simulink model "fullMF"  (R2023b)
settings: Solver=VariableStepAuto  StartTime=0.0  StopTime=3000/fs  RelTol=1e-3
values from neighbouring files (symbols this model uses):
  fs = 16e6    (= 16000000)    [FullMF_startup.m]    (also in MF_startup.m)
  template11 = part11-part21    [FullMF_startup.m]
  template12 = part12-part22    [FullMF_startup.m]
  template13 = part13-part23    [FullMF_startup.m]
  template14 = part14-part24    [FullMF_startup.m]
  template21 = part31+part41    [FullMF_startup.m]
  template22 = part32+part42    [FullMF_startup.m]
  template23 = part33+part43    [FullMF_startup.m]
  template24 = part34+part44    [FullMF_startup.m]
undefined symbols (not defined in the file or in its folder): exp_W1, exp_W2, exp_W3, exp_W4
libraries: hdlBasic x200, hdlDSPIP x20, hdlsllib x1, vmcUtilities x1
(part 2 of 2)

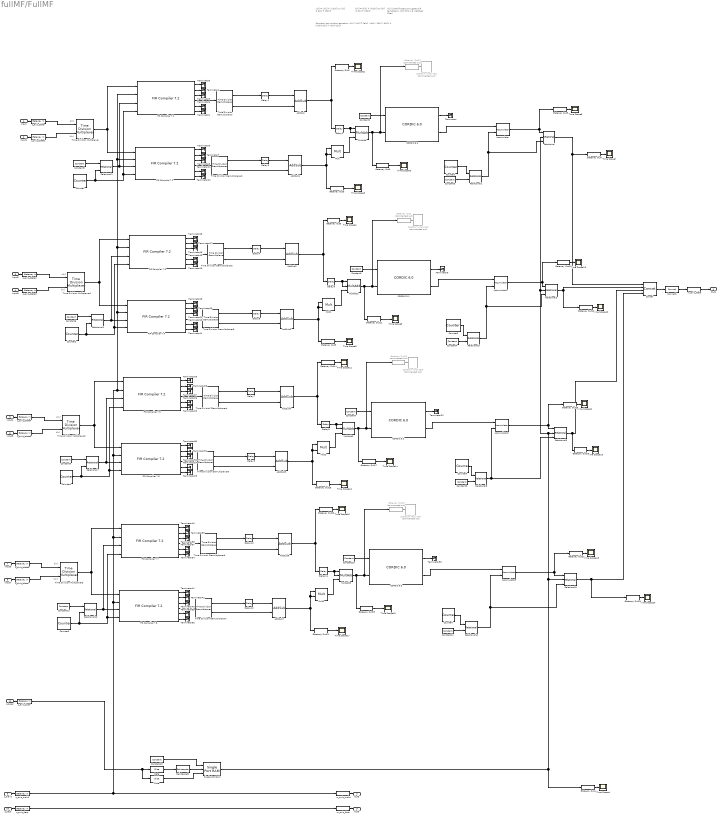
== system fullMF/FullMF ==
  note: a[n]
  note: b[n]
  note: x[n] = xl[n] + j(xq[n])
      | or
      | x[n] = a[n] + j(b[n])
  note: h[n] = hl[n] + j(hq[n])
      | or
      | h[n] = c[n] + j(d[n])
  note: h[n] is the flipped conjugate
      | of a template in x[n]
      | (this is a matched filter)
  note: Complex convolution equation:
      |
      | x[n] * h[n] = ((a[n] * c[n]) - (b[n] * d[n])) + j((a[n]*d[n]) + (b[n]*c[n]))
  note: a[n]
  note: b[n]
  note: a[n]
  note: b[n]
  note: a[n]
  note: b[n]
  Input : Inport
  Input1 : Inport  Port=2
  Input2 : Inport  Port=3
  Input3 : Inport  Port=4
  Input4 : Inport  Port=5
  Input5 : Inport  Port=6
  Input6 : Inport  Port=7
  Input7 : Inport  Port=8
  s_tvalid : Inport  Port=9
  s_tlast : Inport  Port=10
  s_tuser : Inport  Port=11
  Accumulator{,1..3} (4 alike) : hdlBasic/Accumulator  operation=Add  n_bits=64  overflow=Wrap  scale=1  rst=on  hasbypass=off  en=off  latency=1  msb_inp=100  msb=100  lsb=-100  use_behavioral_HDL=on  implementation=Fabric  XmcBlockStatus=1  maskContainerNames=group3  block_type=accum  block_config=sysgen:Accum_config  block_width=566  block_height=845
  AddSub{,2,4,6} (4 alike) : hdlBasic/AddSub  mode=Subtraction  use_carryin=off  use_carryout=off  en=off  latency=1  precision=Full  arith_type=Unsigned  n_bits=16  bin_pt=14  quantization=Truncate  overflow=Wrap  use_behavioral_HDL=off  hw_selection=Fabric  pipelined=off  XmcBlockStatus=1  maskContainerNames=tabcontainer1  block_type=addsub  block_config=sysgen:Addsub_config
  AddSub{1,3,5,7} (4 alike) : hdlBasic/AddSub  mode=Addition  use_carryin=off  use_carryout=off  en=off  latency=1  precision=Full  arith_type=Unsigned  n_bits=16  bin_pt=14  quantization=Truncate  overflow=Wrap  use_behavioral_HDL=off  hw_selection=Fabric  pipelined=off  XmcBlockStatus=1  maskContainerNames=tabcontainer1  block_type=addsub  block_config=sysgen:Addsub_config
  CORDIC 6.{0..3} (4 alike) : hdlDSPIP/CORDIC 6.0   functional_selection=Square_Root  architectural_configuration=Parallel  pipelining_mode=Maximum  data_format=UnsignedInteger  phase_format=Radians  input_width=46  output_width=24  round_mode=Truncate  iterations=0  precision=0  compensation_scaling=No_Scale_Compensation  coarse_rotation=off  aclken=off  aresetn=off  out_tready=off  cartesian_has_tuser=off  cartesian_has_tlast=off  cartesian_tuser_width=1  phase_has_tuser=off  phase_has_tlast=off  phase_tuser_width=1  out_tlast_behv=Null  flow_control=NonBlocking  optimize_goal=Resources  trim_axipin_name=on  simulation_type=hybrid_sim  simulation_model=sysgen:cordic_v6_0  data_path_portlist={'s_axis_cartesian_tdata_imag', 's_axis_cartesian_tdata_real', 's_axis_phase_tdata_phase', 'm_axis_dout_tdata_imag', 'm_axis_dout_tdata_real', 'm_axis_dout_tdata_phase','m_axis_dout_tdata'}  ip_name=CORDIC  ip_version=6.0  dsptool_ready=true  ipcore_usecache=true  ipcore_useipmodelcache=true  wrapper_available=true  port_translation_map={ 'aclken' => 'en', 'aresetn' => 'rst' }  XmcBlockStatus=1  maskContainerNames=group15  block_type=cordic_v6_0  block_config=sysgen:rodinimport_config  block_width=800
  Concat : hdlBasic/Concat  num_inputs=4  XmcBlockStatus=1  maskContainerNames=group1  block_type=concat  block_config=sysgen:Concat_config
  Constant{1..2,7,10} (4 alike) : hdlBasic/Constant  const=1.0  gui_display_data_type=Boolean  arith_type=Boolean  n_bits=16  bin_pt=14  preci_type=Single  exp_width=8  frac_width=24  explicit_period=off  period=1  XmcBlockStatus=1  maskContainerNames=tabcontainer1  block_type=constant  block_config=sysgen:Constant_config
  Constant{3..4,8,11} (4 alike) : hdlBasic/Constant  const=512  gui_display_data_type=Fixed-point  arith_type=Unsigned  n_bits=16  bin_pt=0  preci_type=Single  exp_width=8  frac_width=24  explicit_period=off  period=1  XmcBlockStatus=1  maskContainerNames=tabcontainer1  block_type=constant  block_config=sysgen:Constant_config
  Constant{5..6,9,12} (4 alike) : hdlBasic/Constant  const=1.0  gui_display_data_type=Fixed-point  arith_type=Signed (2's comp)  n_bits=16  bin_pt=14  preci_type=Single  exp_width=8  frac_width=24  explicit_period=off  period=1  XmcBlockStatus=1  maskContainerNames=tabcontainer1  block_type=constant  block_config=sysgen:Constant_config
  Constant13 : hdlBasic/Constant  const=1.0  gui_display_data_type=Fixed-point  arith_type=Unsigned  n_bits=1  bin_pt=0  preci_type=Single  exp_width=8  frac_width=24  explicit_period=off  period=1  XmcBlockStatus=1  maskContainerNames=tabcontainer1  block_type=constant  block_config=sysgen:Constant_config
  Convert1 : hdlBasic/Convert  gui_display_data_type=Fixed-point  arith_type=Signed (2's comp)  n_bits=32  bin_pt=16  float_type=Single  exp_bits=8  fraction_bits=24  quantization=Truncate  overflow=Wrap  en=off  latency=1  pipeline=off  XmcBlockStatus=1  maskContainerNames=group2  block_type=convert  block_config=sysgen:Convert_config  block_width=595  block_height=885
  Counter{,2,4,6} (4 alike) : hdlBasic/Counter  cnt_type=Count limited  cnt_to=1  operation=Up  start_count=0  cnt_by_val=1  arith_type=Unsigned  n_bits=1  bin_pt=0  load_pin=off  rst=off  en=off  explicit_period=Explicit  period=1/(2*fs)  use_behavioral_HDL=off  implementation=Fabric  XmcBlockStatus=1  maskContainerNames=group1  block_type=counter  block_config=sysgen:Counter_config  block_width=531  block_height=1023
  Counter{1,3,5,7} (4 alike) : hdlBasic/Counter  cnt_type=Count limited  cnt_to=512  operation=Up  start_count=0  cnt_by_val=1  arith_type=Unsigned  n_bits=16  bin_pt=0  load_pin=off  rst=off  en=off  explicit_period=Explicit  period=1/fs  use_behavioral_HDL=off  implementation=Fabric  XmcBlockStatus=1  maskContainerNames=group1  block_type=counter  block_config=sysgen:Counter_config  block_width=531  block_height=1023
  Data : hdlBasic/Slice  nbits=15  boolean_output=off  mode=Upper Bit Location + Width  bit1=15  base1=LSB of Input  bit0=16*8-(16*1)  base0=LSB of Input  XmcBlockStatus=1  maskContainerNames=group1  block_type=slice  block_config=sysgen:Slice_config
  Delay{1,3..4,6..7,9..10,12} (8 alike) : hdlBasic/Delay  rst=off  en=off  latency=1  reg_retiming=off  XmcBlockStatus=1  maskContainerNames=group1  block_type=delay  block_config=sysgen:Delay_config
  Delay{2,5,8,11} (4 alike) : hdlBasic/Delay  rst=off  en=off  latency=3  reg_retiming=off  XmcBlockStatus=1  maskContainerNames=group1  block_type=delay  block_config=sysgen:Delay_config
  FIR Compiler 7.1 : hdlDSPIP/FIR Compiler 7.2   coefficientvector=[template11, template21]  coefficient_sets=2  coefficient_reload=off  filter_type=Single_Rate  rate_change_type=Integer  interpolation_rate=1  decimation_rate=1  zero_pack_factor=1  channel_sequence=Basic  number_channels=2  pattern_list='P4-0,P4-1,P4-2,P4-3,P4-4'  number_paths=1  ratespecification=Maximum_Possible  sampleperiod=1  hardwareoversamplingrate=1  coefficient_sign=Signed  quantization=Quantize_Only  coefficient_width=16  bestprecision=off  coefficient_fractional_bits=14  coefficient_structure=Inferred  output_rounding_mode=Full_Precision  output_width=32  filter_architecture=Systolic_Multiply_Accumulate  optimization_goal=Area  optimization_list='None'  data_buffer_type=Automatic  coefficient_buffer_type=Automatic  input_buffer_type=Automatic  output_buffer_type=Automatic  preference_for_other_storage=Automatic  multi_column_support=Automatic  columnconfig='10'  inter_column_pipe_length=4  data_has_tlast=Not_Required  m_data_has_tready=off  s_data_has_fifo=off  s_data_has_tuser=Not_Required  m_data_has_tuser=Not_Required  s_config_sync_mode=On_Vector  s_config_method=By_Channel  num_reload_slots=1  has_aclken=off  has_aresetn=off  reset_data_vector=on  trim_axipin_name=on  simulation_type=hybrid_sim  simulation_model=sysgen:xfirv7_2_cmodel  data_path_portlist={ 's_axis_data_tdata', 'm_axis_data_tdata' }  passband_min=0.0  passband_max=0.5  stopband_min=0.5  stopband_max=1.0  filter_selection=1  gui_behaviour='Sysgen_GUI'  data_sign=Signed  data_width=16  data_fractional_bits=0  data_tuser_width=1  wrapper_available=true  ip_wrap_arbitrary_binary_point=true  ip_name=FIR Compiler  ip_version=7.2  dsptool_ready=true  ipcore_usecache=true  ipcore_useipmodelcache=true  port_translation_map={ 'aclken' => 'en', 'aresetn' => 'rst' }  run_core_at_system_period=true  ipcore_xco_need_fpga_part=true  ipcore_fpga_part=[]  XmcBlockStatus=1  maskContainerNames=tabcontainer1  block_type=fir_compiler_v7_2  block_config=sysgen:rodinimport_config  block_width=820  block_height=600
  FIR Compiler 7.2 : hdlDSPIP/FIR Compiler 7.2   coefficientvector=[template21, template11]  coefficient_sets=2  coefficient_reload=off  filter_type=Single_Rate  rate_change_type=Integer  interpolation_rate=1  decimation_rate=1  zero_pack_factor=1  channel_sequence=Basic  number_channels=2  pattern_list='P4-0,P4-1,P4-2,P4-3,P4-4'  number_paths=1  ratespecification=Maximum_Possible  sampleperiod=1  hardwareoversamplingrate=1  coefficient_sign=Signed  quantization=Quantize_Only  coefficient_width=16  bestprecision=off  coefficient_fractional_bits=14  coefficient_structure=Inferred  output_rounding_mode=Full_Precision  output_width=32  filter_architecture=Systolic_Multiply_Accumulate  optimization_goal=Area  optimization_list='None'  data_buffer_type=Automatic  coefficient_buffer_type=Automatic  input_buffer_type=Automatic  output_buffer_type=Automatic  preference_for_other_storage=Automatic  multi_column_support=Automatic  columnconfig='10'  inter_column_pipe_length=4  data_has_tlast=Not_Required  m_data_has_tready=off  s_data_has_fifo=off  s_data_has_tuser=Not_Required  m_data_has_tuser=Not_Required  s_config_sync_mode=On_Vector  s_config_method=By_Channel  num_reload_slots=1  has_aclken=off  has_aresetn=off  reset_data_vector=on  trim_axipin_name=on  simulation_type=hybrid_sim  simulation_model=sysgen:xfirv7_2_cmodel  data_path_portlist={ 's_axis_data_tdata', 'm_axis_data_tdata' }  passband_min=0.0  passband_max=0.5  stopband_min=0.5  stopband_max=1.0  filter_selection=1  gui_behaviour='Sysgen_GUI'  data_sign=Signed  data_width=16  data_fractional_bits=0  data_tuser_width=1  wrapper_available=true  ip_wrap_arbitrary_binary_point=true  ip_name=FIR Compiler  ip_version=7.2  dsptool_ready=true  ipcore_usecache=true  ipcore_useipmodelcache=true  port_translation_map={ 'aclken' => 'en', 'aresetn' => 'rst' }  run_core_at_system_period=true  ipcore_xco_need_fpga_part=true  ipcore_fpga_part=[]  XmcBlockStatus=1  maskContainerNames=tabcontainer1  block_type=fir_compiler_v7_2  block_config=sysgen:rodinimport_config  block_width=820  block_height=600
  FIR Compiler 7.3 : hdlDSPIP/FIR Compiler 7.2   coefficientvector=[template12, template22]  coefficient_sets=2  coefficient_reload=off  filter_type=Single_Rate  rate_change_type=Integer  interpolation_rate=1  decimation_rate=1  zero_pack_factor=1  channel_sequence=Basic  number_channels=2  pattern_list='P4-0,P4-1,P4-2,P4-3,P4-4'  number_paths=1  ratespecification=Maximum_Possible  sampleperiod=1  hardwareoversamplingrate=1  coefficient_sign=Signed  quantization=Quantize_Only  coefficient_width=16  bestprecision=off  coefficient_fractional_bits=14  coefficient_structure=Inferred  output_rounding_mode=Full_Precision  output_width=35  filter_architecture=Systolic_Multiply_Accumulate  optimization_goal=Area  optimization_list='None'  data_buffer_type=Automatic  coefficient_buffer_type=Automatic  input_buffer_type=Automatic  output_buffer_type=Automatic  preference_for_other_storage=Automatic  multi_column_support=Automatic  columnconfig='100'  inter_column_pipe_length=4  data_has_tlast=Not_Required  m_data_has_tready=off  s_data_has_fifo=off  s_data_has_tuser=Not_Required  m_data_has_tuser=Not_Required  s_config_sync_mode=On_Vector  s_config_method=By_Channel  num_reload_slots=1  has_aclken=off  has_aresetn=off  reset_data_vector=on  trim_axipin_name=on  simulation_type=hybrid_sim  simulation_model=sysgen:xfirv7_2_cmodel  data_path_portlist={ 's_axis_data_tdata', 'm_axis_data_tdata' }  passband_min=0.0  passband_max=0.5  stopband_min=0.5  stopband_max=1.0  filter_selection=1  gui_behaviour='Sysgen_GUI'  data_sign=Signed  data_width=16  data_fractional_bits=0  data_tuser_width=1  wrapper_available=true  ip_wrap_arbitrary_binary_point=true  ip_name=FIR Compiler  ip_version=7.2  dsptool_ready=true  ipcore_usecache=true  ipcore_useipmodelcache=true  port_translation_map={ 'aclken' => 'en', 'aresetn' => 'rst' }  run_core_at_system_period=true  ipcore_xco_need_fpga_part=true  ipcore_fpga_part=[]  XmcBlockStatus=1  maskContainerNames=tabcontainer1  block_type=fir_compiler_v7_2  block_config=sysgen:rodinimport_config  block_width=820  block_height=600
  FIR Compiler 7.4 : hdlDSPIP/FIR Compiler 7.2   coefficientvector=[template22 template12]  coefficient_sets=2  coefficient_reload=off  filter_type=Single_Rate  rate_change_type=Integer  interpolation_rate=1  decimation_rate=1  zero_pack_factor=1  channel_sequence=Basic  number_channels=2  pattern_list='P4-0,P4-1,P4-2,P4-3,P4-4'  number_paths=1  ratespecification=Maximum_Possible  sampleperiod=1  hardwareoversamplingrate=1  coefficient_sign=Signed  quantization=Quantize_Only  coefficient_width=16  bestprecision=off  coefficient_fractional_bits=14  coefficient_structure=Inferred  output_rounding_mode=Full_Precision  output_width=31  filter_architecture=Systolic_Multiply_Accumulate  optimization_goal=Area  optimization_list='None'  data_buffer_type=Automatic  coefficient_buffer_type=Automatic  input_buffer_type=Automatic  output_buffer_type=Automatic  preference_for_other_storage=Automatic  multi_column_support=Automatic  columnconfig='117'  inter_column_pipe_length=4  data_has_tlast=Not_Required  m_data_has_tready=off  s_data_has_fifo=off  s_data_has_tuser=Not_Required  m_data_has_tuser=Not_Required  s_config_sync_mode=On_Vector  s_config_method=By_Channel  num_reload_slots=1  has_aclken=off  has_aresetn=off  reset_data_vector=on  trim_axipin_name=on  simulation_type=hybrid_sim  simulation_model=sysgen:xfirv7_2_cmodel  data_path_portlist={ 's_axis_data_tdata', 'm_axis_data_tdata' }  passband_min=0.0  passband_max=0.5  stopband_min=0.5  stopband_max=1.0  filter_selection=1  gui_behaviour='Sysgen_GUI'  data_sign=Signed  data_width=16  data_fractional_bits=0  data_tuser_width=1  wrapper_available=true  ip_wrap_arbitrary_binary_point=true  ip_name=FIR Compiler  ip_version=7.2  dsptool_ready=true  ipcore_usecache=true  ipcore_useipmodelcache=true  port_translation_map={ 'aclken' => 'en', 'aresetn' => 'rst' }  run_core_at_system_period=true  ipcore_xco_need_fpga_part=true  ipcore_fpga_part=[]  XmcBlockStatus=1  maskContainerNames=tabcontainer1  block_type=fir_compiler_v7_2  block_config=sysgen:rodinimport_config  block_width=820  block_height=600
  FIR Compiler 7.5 : hdlDSPIP/FIR Compiler 7.2   coefficientvector=[template13, template23]  coefficient_sets=2  coefficient_reload=off  filter_type=Single_Rate  rate_change_type=Integer  interpolation_rate=1  decimation_rate=1  zero_pack_factor=1  channel_sequence=Basic  number_channels=2  pattern_list='P4-0,P4-1,P4-2,P4-3,P4-4'  number_paths=1  ratespecification=Maximum_Possible  sampleperiod=1  hardwareoversamplingrate=1  coefficient_sign=Signed  quantization=Quantize_Only  coefficient_width=16  bestprecision=off  coefficient_fractional_bits=14  coefficient_structure=Inferred  output_rounding_mode=Full_Precision  output_width=31  filter_architecture=Systolic_Multiply_Accumulate  optimization_goal=Area  optimization_list='None'  data_buffer_type=Automatic  coefficient_buffer_type=Automatic  input_buffer_type=Automatic  output_buffer_type=Automatic  preference_for_other_storage=Automatic  multi_column_support=Automatic  columnconfig='117'  inter_column_pipe_length=4  data_has_tlast=Not_Required  m_data_has_tready=off  s_data_has_fifo=off  s_data_has_tuser=Not_Required  m_data_has_tuser=Not_Required  s_config_sync_mode=On_Vector  s_config_method=By_Channel  num_reload_slots=1  has_aclken=off  has_aresetn=off  reset_data_vector=on  trim_axipin_name=on  simulation_type=hybrid_sim  simulation_model=sysgen:xfirv7_2_cmodel  data_path_portlist={ 's_axis_data_tdata', 'm_axis_data_tdata' }  passband_min=0.0  passband_max=0.5  stopband_min=0.5  stopband_max=1.0  filter_selection=1  gui_behaviour='Sysgen_GUI'  data_sign=Signed  data_width=16  data_fractional_bits=0  data_tuser_width=1  wrapper_available=true  ip_wrap_arbitrary_binary_point=true  ip_name=FIR Compiler  ip_version=7.2  dsptool_ready=true  ipcore_usecache=true  ipcore_useipmodelcache=true  port_translation_map={ 'aclken' => 'en', 'aresetn' => 'rst' }  run_core_at_system_period=true  ipcore_xco_need_fpga_part=true  ipcore_fpga_part=[]  XmcBlockStatus=1  maskContainerNames=tabcontainer1  block_type=fir_compiler_v7_2  block_config=sysgen:rodinimport_config  block_width=820  block_height=600
  FIR Compiler 7.6 : hdlDSPIP/FIR Compiler 7.2   coefficientvector=[template23, template13]  coefficient_sets=2  coefficient_reload=off  filter_type=Single_Rate  rate_change_type=Integer  interpolation_rate=1  decimation_rate=1  zero_pack_factor=1  channel_sequence=Basic  number_channels=2  pattern_list='P4-0,P4-1,P4-2,P4-3,P4-4'  number_paths=1  ratespecification=Maximum_Possible  sampleperiod=1  hardwareoversamplingrate=1  coefficient_sign=Signed  quantization=Quantize_Only  coefficient_width=16  bestprecision=off  coefficient_fractional_bits=14  coefficient_structure=Inferred  output_rounding_mode=Full_Precision  output_width=31  filter_architecture=Systolic_Multiply_Accumulate  optimization_goal=Area  optimization_list='None'  data_buffer_type=Automatic  coefficient_buffer_type=Automatic  input_buffer_type=Automatic  output_buffer_type=Automatic  preference_for_other_storage=Automatic  multi_column_support=Automatic  columnconfig='117'  inter_column_pipe_length=4  data_has_tlast=Not_Required  m_data_has_tready=off  s_data_has_fifo=off  s_data_has_tuser=Not_Required  m_data_has_tuser=Not_Required  s_config_sync_mode=On_Vector  s_config_method=By_Channel  num_reload_slots=1  has_aclken=off  has_aresetn=off  reset_data_vector=on  trim_axipin_name=on  simulation_type=hybrid_sim  simulation_model=sysgen:xfirv7_2_cmodel  data_path_portlist={ 's_axis_data_tdata', 'm_axis_data_tdata' }  passband_min=0.0  passband_max=0.5  stopband_min=0.5  stopband_max=1.0  filter_selection=1  gui_behaviour='Sysgen_GUI'  data_sign=Signed  data_width=16  data_fractional_bits=0  data_tuser_width=1  wrapper_available=true  ip_wrap_arbitrary_binary_point=true  ip_name=FIR Compiler  ip_version=7.2  dsptool_ready=true  ipcore_usecache=true  ipcore_useipmodelcache=true  port_translation_map={ 'aclken' => 'en', 'aresetn' => 'rst' }  run_core_at_system_period=true  ipcore_xco_need_fpga_part=true  ipcore_fpga_part=[]  XmcBlockStatus=1  maskContainerNames=tabcontainer1  block_type=fir_compiler_v7_2  block_config=sysgen:rodinimport_config  block_width=820  block_height=600
  FIR Compiler 7.7 : hdlDSPIP/FIR Compiler 7.2   coefficientvector=[template14, template24]  coefficient_sets=2  coefficient_reload=off  filter_type=Single_Rate  rate_change_type=Integer  interpolation_rate=1  decimation_rate=1  zero_pack_factor=1  channel_sequence=Basic  number_channels=2  pattern_list='P4-0,P4-1,P4-2,P4-3,P4-4'  number_paths=1  ratespecification=Maximum_Possible  sampleperiod=1  hardwareoversamplingrate=1  coefficient_sign=Signed  quantization=Quantize_Only  coefficient_width=16  bestprecision=off  coefficient_fractional_bits=14  coefficient_structure=Inferred  output_rounding_mode=Full_Precision  output_width=31  filter_architecture=Systolic_Multiply_Accumulate  optimization_goal=Area  optimization_list='None'  data_buffer_type=Automatic  coefficient_buffer_type=Automatic  input_buffer_type=Automatic  output_buffer_type=Automatic  preference_for_other_storage=Automatic  multi_column_support=Automatic  columnconfig='117'  inter_column_pipe_length=4  data_has_tlast=Not_Required  m_data_has_tready=off  s_data_has_fifo=off  s_data_has_tuser=Not_Required  m_data_has_tuser=Not_Required  s_config_sync_mode=On_Vector  s_config_method=By_Channel  num_reload_slots=1  has_aclken=off  has_aresetn=off  reset_data_vector=on  trim_axipin_name=on  simulation_type=hybrid_sim  simulation_model=sysgen:xfirv7_2_cmodel  data_path_portlist={ 's_axis_data_tdata', 'm_axis_data_tdata' }  passband_min=0.0  passband_max=0.5  stopband_min=0.5  stopband_max=1.0  filter_selection=1  gui_behaviour='Sysgen_GUI'  data_sign=Signed  data_width=16  data_fractional_bits=0  data_tuser_width=1  wrapper_available=true  ip_wrap_arbitrary_binary_point=true  ip_name=FIR Compiler  ip_version=7.2  dsptool_ready=true  ipcore_usecache=true  ipcore_useipmodelcache=true  port_translation_map={ 'aclken' => 'en', 'aresetn' => 'rst' }  run_core_at_system_period=true  ipcore_xco_need_fpga_part=true  ipcore_fpga_part=[]  XmcBlockStatus=1  maskContainerNames=tabcontainer1  block_type=fir_compiler_v7_2  block_config=sysgen:rodinimport_config  block_width=820  block_height=600
  FIR Compiler 7.8 : hdlDSPIP/FIR Compiler 7.2   coefficientvector=[template24, template14]  coefficient_sets=2  coefficient_reload=off  filter_type=Single_Rate  rate_change_type=Integer  interpolation_rate=1  decimation_rate=1  zero_pack_factor=1  channel_sequence=Basic  number_channels=2  pattern_list='P4-0,P4-1,P4-2,P4-3,P4-4'  number_paths=1  ratespecification=Maximum_Possible  sampleperiod=1  hardwareoversamplingrate=1  coefficient_sign=Signed  quantization=Quantize_Only  coefficient_width=16  bestprecision=off  coefficient_fractional_bits=14  coefficient_structure=Inferred  output_rounding_mode=Full_Precision  output_width=31  filter_architecture=Systolic_Multiply_Accumulate  optimization_goal=Area  optimization_list='None'  data_buffer_type=Automatic  coefficient_buffer_type=Automatic  input_buffer_type=Automatic  output_buffer_type=Automatic  preference_for_other_storage=Automatic  multi_column_support=Automatic  columnconfig='117'  inter_column_pipe_length=4  data_has_tlast=Not_Required  m_data_has_tready=off  s_data_has_fifo=off  s_data_has_tuser=Not_Required  m_data_has_tuser=Not_Required  s_config_sync_mode=On_Vector  s_config_method=By_Channel  num_reload_slots=1  has_aclken=off  has_aresetn=off  reset_data_vector=on  trim_axipin_name=on  simulation_type=hybrid_sim  simulation_model=sysgen:xfirv7_2_cmodel  data_path_portlist={ 's_axis_data_tdata', 'm_axis_data_tdata' }  passband_min=0.0  passband_max=0.5  stopband_min=0.5  stopband_max=1.0  filter_selection=1  gui_behaviour='Sysgen_GUI'  data_sign=Signed  data_width=16  data_fractional_bits=0  data_tuser_width=1  wrapper_available=true  ip_wrap_arbitrary_binary_point=true  ip_name=FIR Compiler  ip_version=7.2  dsptool_ready=true  ipcore_usecache=true  ipcore_useipmodelcache=true  port_translation_map={ 'aclken' => 'en', 'aresetn' => 'rst' }  run_core_at_system_period=true  ipcore_xco_need_fpga_part=true  ipcore_fpga_part=[]  XmcBlockStatus=1  maskContainerNames=tabcontainer1  block_type=fir_compiler_v7_2  block_config=sysgen:rodinimport_config  block_width=820  block_height=600
  Gateway Out{1,10,13,19} (4 alike) : hdlBasic/Gateway Out  Commented=on  inherit_from_input=off  hdl_port=off  rows=1  columns=1  UseAsDAC=off  DACChannel='1'  interface=None  automatic_assignment=on  address_offset=hex2dec('00')  intf_name=''  intf_description=''  timing_constraint=None  locs_specified=off  LOCs={}  io_standard={}  XmcBlockStatus=1  maskContainerNames=group4  block_type=gatewayout  block_config=sysgen:gateway_out_config  block_width_w=590  block_height_w=620  block_width=620  block_height=750
  Gateway Out{2..9,11..12,14..18,20..25} (21 alike) : hdlBasic/Gateway Out  inherit_from_input=off  hdl_port=off  rows=1  columns=1  UseAsDAC=off  DACChannel='1'  interface=None  automatic_assignment=on  address_offset=hex2dec('00')  intf_name=''  intf_description=''  timing_constraint=None  locs_specified=off  LOCs={}  io_standard={}  XmcBlockStatus=1  maskContainerNames=group4  block_type=gatewayout  block_config=sysgen:gateway_out_config  block_width_w=590  block_height_w=620  block_width=620  block_height=750
  Mult{,1..3} (4 alike) : hdlBasic/Mult  precision=Full  arith_type="Signed  (2's comp)"  n_bits=16  bin_pt=14  quantization=Truncate  overflow=Wrap  en=off  latency=3  use_behavioral_HDL=off  opt=Speed  use_embedded=on  optimum_pipeline=off  pipeline=on  use_rpm=on  placement_style=Triangular  XmcBlockStatus=1  maskContainerNames=group1  block_type=mult  block_config=sysgen:Mult_config  block_width=598  block_height=876
  MultAdd{,1..3} (4 alike) : hdlBasic/MultAdd  mode=Addition  en=off  latency=0  precision=User Defined  arith_type=Unsigned  n_bits=48  bin_pt=0  XmcBlockStatus=1  maskContainerNames=tabcontainer1  block_type=multadd  block_config=sysgen:MultAdd_config
  Reinterpret2 : hdlBasic/Reinterpret  force_arith_type=on  arith_type=Unsigned  force_bin_pt=on  bin_pt=5  XmcBlockStatus=1  maskContainerNames=group1  block_type=reinterpret  block_config=sysgen:Reinterpret_config
  Relational{,3,6,9} (4 alike) : hdlBasic/Relational  mode=a>b  op_type=Bool  en=on  latency=1  XmcBlockStatus=1  maskContainerNames=tabcontainer1  block_type=relational  block_config=sysgen:Relational_config
  Relational{1..2,4..5,7..8,10..11} (8 alike) : hdlBasic/Relational  mode=a=b  op_type=Bool  en=off  latency=1  XmcBlockStatus=1  maskContainerNames=tabcontainer1  block_type=relational  block_config=sysgen:Relational_config
  Single Port RAM : hdlBasic/Single Port RAM  depth=2  initVector=[0 0]  distributed_mem=Distributed memory  write_mode=Read After Write  rst=off  init_reg=0  en=off  optimize_latency=on  latency=1  optimize=Area  dbl_ovrd=off  simulation_type=fast_sim  XmcBlockStatus=1  maskContainerNames=tabcontainer1  block_type=spram  block_config=sysgen:SPRAM_config
  Spectrum Analyzer{1..4} (4 alike) : SpectrumAnalyzer  Commented=on  SampleRate=16000000  AxesScaling=Manual  Span=16000000  StartFrequency=-8000000  StopFrequency=8000000  AveragingMethod=Exponential  YLimits=[-85.389381881293900278,31.375193648210043307]  DefaultConfigurationName=spbscopes.SpectrumAnalyzerBlockCfg  IsFrequencyInputMode=0  FrequencyVectorPort=0  FrequencyVectorFromPort=0  FrequencyInputRBWPort=0  FrequencyInputRBWFromPort=0
  Terminator{,1..43} (44 alike) : Terminator
  Time Scope{1..21} (21 alike) : Scope
  Time Division Demultiplexer{,1..7} (8 alike) : hdlBasic/Time Division Demultiplexer  frame_pattern=[1 1]  impl_style=Multiple Channel  vin=off  explicit_period=off  period=1  XmcBlockStatus=1  maskContainerNames=group2  block_type=tdd  block_config=sysgen:TDD_config
  Time Division Multiplexer{,1..3} (4 alike) : hdlBasic/Time Division Multiplexer  inputs=2  vin=off  Optimization=Resource  explicit_period=off  period=1  XmcBlockStatus=1  maskContainerNames=group3  block_type=tdm  block_config=sysgen:TDM_config
  Write : hdlBasic/Slice  nbits=1  boolean_output=on  mode=Upper Bit Location + Width  bit1=0  base1=LSB of Input  bit0=16*8-(16*1)  base0=LSB of Input  XmcBlockStatus=1  maskContainerNames=group1  block_type=slice  block_config=sysgen:Slice_config
  m_axis_tdata : hdlBasic/Gateway Out  inherit_from_input=on  hdl_port=on  rows=1  columns=1  UseAsDAC=off  DACChannel='1'  interface=None  automatic_assignment=on  address_offset=hex2dec('00')  intf_name=''  intf_description=''  timing_constraint=None  locs_specified=off  LOCs={}  io_standard={}  XmcBlockStatus=1  maskContainerNames=group4  block_type=gatewayout  block_config=sysgen:gateway_out_config  block_width_w=590  block_height_w=620  block_width=620  block_height=750
  m_axis_tlast : hdlBasic/Gateway Out  inherit_from_input=on  hdl_port=on  rows=1  columns=1  UseAsDAC=off  DACChannel='1'  interface=None  automatic_assignment=on  address_offset=hex2dec('00')  intf_name=''  intf_description=''  timing_constraint=None  locs_specified=off  LOCs={}  io_standard={}  XmcBlockStatus=1  maskContainerNames=group4  block_type=gatewayout  block_config=sysgen:gateway_out_config  block_width_w=590  block_height_w=620  block_width=620  block_height=750
  m_axis_tvalid : hdlBasic/Gateway Out  inherit_from_input=on  hdl_port=on  rows=1  columns=1  UseAsDAC=off  DACChannel='1'  interface=None  automatic_assignment=on  address_offset=hex2dec('00')  intf_name=''  intf_description=''  timing_constraint=None  locs_specified=off  LOCs={}  io_standard={}  XmcBlockStatus=1  maskContainerNames=group4  block_type=gatewayout  block_config=sysgen:gateway_out_config  block_width_w=590  block_height_w=620  block_width=620  block_height=750
  s_axis_tdata{,1..7} (8 alike) : hdlBasic/Gateway In  gui_display_data_type=Fixed-point  arith_type=Signed (2's comp)  n_bits=16  bin_pt=14  preci_type=Single  exp_width=8  frac_width=24  rows=1  columns=1  quantization="Round  (unbiased: +/- Inf)"  overflow=Saturate  period=1/fs  UseAsADC=off  ADCChannel='1'  interface=None  automatic_assignment=on  address_offset=hex2dec('00')  intf_name=''  intf_description=''  default_value=0  timing_constraint=None  locs_specified=off  LOCs={}  io_standard={}  inherit_from_input=off  hdl_port=on  XmcBlockStatus=1  maskContainerNames=group4  block_type=gatewayin  block_config=sysgen:gateway_in_config  block_width_w=590  block_height_w=620  block_width=640  block_height=850
  s_axis_tlast : hdlBasic/Gateway In  gui_display_data_type=Boolean  arith_type=Boolean  n_bits=16  bin_pt=14  preci_type=Single  exp_width=8  frac_width=24  rows=1  columns=1  quantization="Round  (unbiased: +/- Inf)"  overflow=Saturate  period=1/fs  UseAsADC=off  ADCChannel='1'  interface=None  automatic_assignment=on  address_offset=hex2dec('00')  intf_name=''  intf_description=''  default_value=0  timing_constraint=None  locs_specified=off  LOCs={}  io_standard={}  inherit_from_input=off  hdl_port=on  XmcBlockStatus=1  maskContainerNames=group4  block_type=gatewayin  block_config=sysgen:gateway_in_config  block_width_w=590  block_height_w=620  block_width=640  block_height=850
  s_axis_tuser : hdlBasic/Gateway In  gui_display_data_type=Fixed-point  arith_type=Unsigned  n_bits=16  bin_pt=0  preci_type=Single  exp_width=8  frac_width=24  rows=1  columns=1  quantization="Round  (unbiased: +/- Inf)"  overflow=Saturate  period=1/fs  UseAsADC=off  ADCChannel='1'  interface=None  automatic_assignment=on  address_offset=hex2dec('00')  intf_name=''  intf_description=''  default_value=0  timing_constraint=None  locs_specified=off  LOCs={}  io_standard={}  inherit_from_input=off  hdl_port=on  XmcBlockStatus=1  maskContainerNames=group4  block_type=gatewayin  block_config=sysgen:gateway_in_config  block_width_w=590  block_height_w=620  block_width=640  block_height=850
  s_axis_tvalid : hdlBasic/Gateway In  gui_display_data_type=Boolean  arith_type=Boolean  n_bits=16  bin_pt=14  preci_type=Single  exp_width=8  frac_width=24  rows=1  columns=1  quantization="Round  (unbiased: +/- Inf)"  overflow=Saturate  period=1/fs  UseAsADC=off  ADCChannel='1'  interface=None  automatic_assignment=on  address_offset=hex2dec('00')  intf_name=''  intf_description=''  default_value=0  timing_constraint=None  locs_specified=off  LOCs={}  io_standard={}  inherit_from_input=off  hdl_port=on  XmcBlockStatus=1  maskContainerNames=group4  block_type=gatewayin  block_config=sysgen:gateway_in_config  block_width_w=590  block_height_w=620  block_width=640  block_height=850
  Out1 : Outport
  Out5 : Outport  Port=2
  Out6 : Outport  Port=3
  wires:
  s_axis_tvalid/1 -> FIR Compiler 7.1/2, FIR Compiler 7.2/2, FIR Compiler 7.3/2, FIR Compiler 7.4/2, FIR Compiler 7.5/2, FIR Compiler 7.6/2, FIR Compiler 7.7/2, FIR Compiler 7.8/2, m_axis_tvalid/1
  CORDIC 6.2/1 -> Terminator22/1
  Time Division Multiplexer1/1 -> FIR Compiler 7.4/1, FIR Compiler 7.3/1
  Counter1/1 -> Relational2/1
  m_axis_tlast/1 -> Out6/1
  s_axis_tdata/1 -> Time Division Multiplexer/1
  Time Division Multiplexer2/1 -> FIR Compiler 7.6/1, FIR Compiler 7.5/1
  s_tvalid/1 -> s_axis_tvalid/1
  AddSub/1 -> Delay2/1, Gateway Out2/1
  FIR Compiler 7.4/1 -> Terminator19/1
  MultAdd2/1 -> Gateway Out13/1, CORDIC 6.2/2, Gateway Out17/1
  Time Division Demultiplexer2/1 -> Delay4/1
  MultAdd/1 -> Gateway Out10/1, CORDIC 6.0/2, Gateway Out6/1
  FIR Compiler 7.7/3 -> Terminator38/1
  FIR Compiler 7.2/3 -> Terminator8/1
  s_tlast/1 -> s_axis_tlast/1
  CORDIC 6.1/2 -> Accumulator1/1
  Constant6/1 -> Relational4/1
  Single Port RAM/1 -> Gateway Out4/1, Relational9/2, Relational/2, Relational3/2, Relational6/2
  Delay9/1 -> AddSub5/1
  Gateway Out20/1 -> Time Scope16/1
  Delay12/1 -> AddSub7/1
  FIR Compiler 7.8/6 -> Terminator36/1
  s_axis_tdata1/1 -> Time Division Multiplexer/2
  Constant8/1 -> Relational8/2
  s_axis_tdata5/1 -> Time Division Multiplexer2/2
  Counter2/1 -> FIR Compiler 7.4/4, FIR Compiler 7.3/4, Relational4/2
  FIR Compiler 7.5/1 -> Terminator29/1
  FIR Compiler 7.1/5 -> Terminator2/1
  Relational/1 -> Concat/1, Gateway Out7/1
  CORDIC 6.0/2 -> Accumulator/1
  FIR Compiler 7.3/5 -> Terminator15/1
  Constant2/1 -> CORDIC 6.0/1
  FIR Compiler 7.8/5 -> Terminator35/1
  Delay11/1 -> MultAdd3/2, MultAdd3/1
  AddSub1/1 -> Mult/2, Mult/1, Gateway Out3/1
  FIR Compiler 7.6/2 -> Terminator31/1
  Relational9/1 -> Concat/4, Gateway Out24/1
  AddSub7/1 -> Mult3/2, Mult3/1, Gateway Out21/1
  Counter4/1 -> FIR Compiler 7.6/4, FIR Compiler 7.5/4, Relational7/2
  Time Division Demultiplexer1/1 -> Delay3/1
  AddSub5/1 -> Mult2/2, Mult2/1, Gateway Out15/1
  Delay1/1 -> AddSub/1
  AddSub3/1 -> Mult1/2, Mult1/1, Gateway Out8/1
  FIR Compiler 7.7/2 -> Terminator39/1
  FIR Compiler 7.4/5 -> Terminator13/1
  FIR Compiler 7.3/4 -> Time Division Demultiplexer2/1
  Input4/1 -> s_axis_tdata4/1
  MultAdd3/1 -> Gateway Out19/1, CORDIC 6.3/2, Gateway Out23/1
  s_axis_tuser/1 -> Data/1, Write/1
  Counter7/1 -> Relational11/1
  s_axis_tdata6/1 -> Time Division Multiplexer3/1
  Counter/1 -> FIR Compiler 7.2/4, FIR Compiler 7.1/4, Relational1/2
  Gateway Out6/1 -> Time Scope6/1
  CORDIC 6.0/1 -> Terminator/1
  Time Division Demultiplexer7/2 -> AddSub7/2
  Reinterpret2/1 -> Single Port RAM/2
  Gateway Out2/1 -> Time Scope2/1
  Delay5/1 -> MultAdd1/2, MultAdd1/1
  Gateway Out8/1 -> Time Scope5/1
  FIR Compiler 7.1/4 -> Time Division Demultiplexer/1
  Relational7/1 -> FIR Compiler 7.6/3, FIR Compiler 7.5/3
  FIR Compiler 7.4/2 -> Terminator20/1
  Time Division Demultiplexer4/2 -> AddSub4/2
  Delay8/1 -> MultAdd2/2, MultAdd2/1
  Relational3/1 -> Concat/2, Gateway Out12/1
  FIR Compiler 7.4/3 -> Terminator21/1
  AddSub2/1 -> Delay5/1, Gateway Out5/1
  FIR Compiler 7.2/6 -> Terminator12/1
  CORDIC 6.1/1 -> Terminator9/1
  Gateway Out18/1 -> Time Scope15/1
  Relational10/1 -> FIR Compiler 7.8/3, FIR Compiler 7.7/3
  Input6/1 -> s_axis_tdata6/1
  FIR Compiler 7.1/6 -> Terminator1/1
  Input7/1 -> s_axis_tdata7/1
  Time Division Demultiplexer5/2 -> AddSub5/2
  Delay3/1 -> AddSub1/1
  FIR Compiler 7.4/6 -> Terminator14/1
  s_axis_tdata3/1 -> Time Division Multiplexer1/2
  Gateway Out15/1 -> Time Scope12/1
  Constant12/1 -> Relational10/1
  FIR Compiler 7.2/5 -> Terminator11/1
  Time Division Demultiplexer/2 -> AddSub/2
  Time Division Demultiplexer1/2 -> AddSub1/2
  FIR Compiler 7.3/1 -> Terminator18/1
  Counter5/1 -> Relational8/1
  Constant4/1 -> Relational5/2
  Relational4/1 -> FIR Compiler 7.4/3, FIR Compiler 7.3/3
  FIR Compiler 7.7/4 -> Time Division Demultiplexer6/1
  Delay7/1 -> AddSub4/1
  Write/1 -> Single Port RAM/3
  Time Division Demultiplexer3/1 -> Delay6/1
  MultAdd1/1 -> Gateway Out1/1, CORDIC 6.1/2, Gateway Out11/1
  s_axis_tdata2/1 -> Time Division Multiplexer1/1
  FIR Compiler 7.4/4 -> Time Division Demultiplexer3/1
  FIR Compiler 7.3/2 -> Terminator17/1
  Delay2/1 -> MultAdd/2, MultAdd/1
  AddSub4/1 -> Delay8/1, Gateway Out14/1
  FIR Compiler 7.5/5 -> Terminator26/1
  Gateway Out11/1 -> Time Scope9/1
  Gateway Out1/1 -> Spectrum Analyzer2/1
  Gateway Out12/1 -> Time Scope10/1
  FIR Compiler 7.3/6 -> Terminator10/1
  Time Division Multiplexer3/1 -> FIR Compiler 7.8/1, FIR Compiler 7.7/1
  Counter3/1 -> Relational5/1
  FIR Compiler 7.3/3 -> Terminator16/1
  Delay6/1 -> AddSub3/1
  Time Division Demultiplexer3/2 -> AddSub3/2
  FIR Compiler 7.1/3 -> Terminator3/1
  FIR Compiler 7.1/2 -> Terminator4/1
  Relational6/1 -> Gateway Out18/1, Concat/3
  Time Division Multiplexer/1 -> FIR Compiler 7.2/1, FIR Compiler 7.1/1
  Counter6/1 -> FIR Compiler 7.8/4, FIR Compiler 7.7/4, Relational10/2
  FIR Compiler 7.7/1 -> Terminator40/1
  AddSub6/1 -> Delay11/1, Gateway Out20/1
  Relational1/1 -> FIR Compiler 7.2/3, FIR Compiler 7.1/3
  Input1/1 -> s_axis_tdata1/1
  Constant11/1 -> Relational11/2
  s_axis_tdata4/1 -> Time Division Multiplexer2/1
  Time Division Demultiplexer7/1 -> Delay12/1
  Constant10/1 -> CORDIC 6.3/1
  FIR Compiler 7.6/1 -> Terminator30/1
  FIR Compiler 7.8/4 -> Time Division Demultiplexer7/1
  Time Division Demultiplexer/1 -> Delay1/1
  FIR Compiler 7.7/6 -> Terminator34/1
  Constant1/1 -> CORDIC 6.1/1
  Gateway Out23/1 -> Time Scope19/1
  Gateway Out19/1 -> Spectrum Analyzer4/1
  Constant7/1 -> CORDIC 6.2/1
  Input2/1 -> s_axis_tdata2/1
  Time Division Demultiplexer6/1 -> Delay10/1
  Time Division Demultiplexer2/2 -> AddSub2/2
  Gateway Out5/1 -> Time Scope1/1
  FIR Compiler 7.2/2 -> Terminator7/1
  s_axis_tdata7/1 -> Time Division Multiplexer3/2
  Gateway Out7/1 -> Time Scope7/1
  FIR Compiler 7.6/5 -> Terminator24/1
  Constant13/1 -> Single Port RAM/1
  s_axis_tlast/1 -> m_axis_tlast/1
  Gateway Out10/1 -> Spectrum Analyzer1/1
  Time Division Demultiplexer6/2 -> AddSub6/2
  Delay4/1 -> AddSub2/1
  Constant9/1 -> Relational7/1
  Time Division Demultiplexer4/1 -> Delay7/1
  Mult1/1 -> MultAdd1/3
  Gateway Out3/1 -> Time Scope3/1
  FIR Compiler 7.2/4 -> Time Division Demultiplexer1/1
  CORDIC 6.3/1 -> Terminator33/1
  FIR Compiler 7.8/1 -> Terminator41/1
  FIR Compiler 7.6/4 -> Time Division Demultiplexer5/1
  Data/1 -> Reinterpret2/1
  FIR Compiler 7.5/2 -> Terminator28/1
  Constant3/1 -> Relational2/2
  Time Division Demultiplexer5/1 -> Delay9/1
  Input/1 -> s_axis_tdata/1
  Mult2/1 -> MultAdd2/3
  m_axis_tvalid/1 -> Out5/1
  Gateway Out24/1 -> Time Scope20/1
  Gateway Out13/1 -> Spectrum Analyzer3/1
  FIR Compiler 7.5/6 -> Terminator23/1
  Mult/1 -> MultAdd/3
  CORDIC 6.3/2 -> Accumulator3/1
  Constant5/1 -> Relational1/1
  CORDIC 6.2/2 -> Accumulator2/1
  FIR Compiler 7.5/4 -> Time Division Demultiplexer4/1
  FIR Compiler 7.6/3 -> Terminator32/1
  FIR Compiler 7.6/6 -> Terminator25/1
  Gateway Out21/1 -> Time Scope17/1
  Gateway Out14/1 -> Time Scope11/1
  Gateway Out17/1 -> Time Scope14/1
  FIR Compiler 7.7/5 -> Terminator37/1
  FIR Compiler 7.8/3 -> Terminator43/1
  FIR Compiler 7.8/2 -> Terminator42/1
  Delay10/1 -> AddSub6/1
  Mult3/1 -> MultAdd3/3
  FIR Compiler 7.5/3 -> Terminator27/1
  FIR Compiler 7.2/1 -> Terminator6/1
  FIR Compiler 7.1/1 -> Terminator5/1
  Input5/1 -> s_axis_tdata5/1
  Input3/1 -> s_axis_tdata3/1
  s_tuser/1 -> s_axis_tuser/1
  Concat/1 -> Convert1/1
  Convert1/1 -> m_axis_tdata/1
  m_axis_tdata/1 -> Out1/1
  Relational2/1 -> Relational/3, Accumulator/2
  Accumulator/1 -> Relational/1, Gateway Out9/1
  Accumulator1/1 -> Relational3/1, Gateway Out16/1
  Relational5/1 -> Relational3/3, Accumulator1/2
  Accumulator2/1 -> Relational6/1, Gateway Out25/1
  Relational8/1 -> Relational6/3, Accumulator2/2
  Accumulator3/1 -> Relational9/1, Gateway Out22/1
  Relational11/1 -> Relational9/3, Accumulator3/2
  Gateway Out22/1 -> Time Scope18/1
  Gateway Out25/1 -> Time Scope21/1
  Gateway Out16/1 -> Time Scope13/1
  Gateway Out9/1 -> Time Scope8/1
  Gateway Out4/1 -> Time Scope4/1

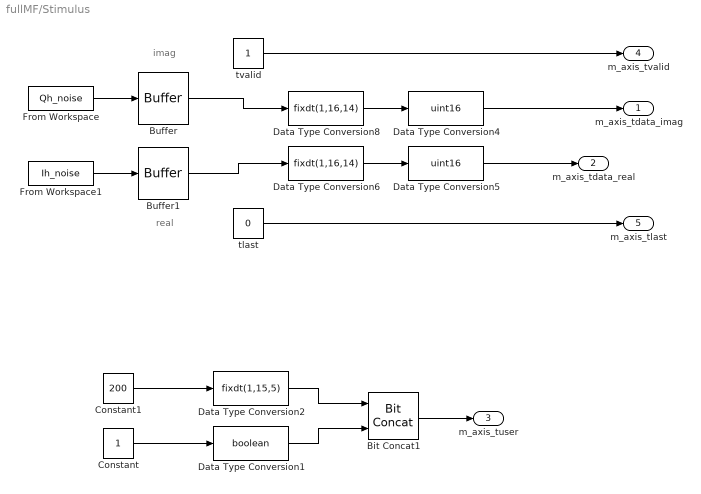
== system fullMF/Stimulus ==
  note: real
  note: imag
  Bit Concat1 : hdlsllib/Logic and Bit Operations/Bit Concat  numInputs=2
  Buffer : Buffer  N=1  OutputFrames=off
  Buffer1 : Buffer  N=1  OutputFrames=off
  Constant : Constant  SampleTime=1/fs
  Constant1 : Constant  Value=200  SampleTime=1/fs
  Data Type Conversion1 : DataTypeConversion  OutDataTypeStr=boolean  RndMeth=Floor
  Data Type Conversion2 : DataTypeConversion  OutDataTypeStr=fixdt(1,15,5)  RndMeth=Floor
  Data Type Conversion4 : DataTypeConversion  OutDataTypeStr=uint16  ConvertRealWorld=Stored Integer (SI)  RndMeth=Floor
  Data Type Conversion5 : DataTypeConversion  OutDataTypeStr=uint16  ConvertRealWorld=Stored Integer (SI)  RndMeth=Floor
  Data Type Conversion6 : DataTypeConversion  OutDataTypeStr=fixdt(1,16,14)  RndMeth=Floor
  Data Type Conversion8 : DataTypeConversion  OutDataTypeStr=fixdt(1,16,14)  RndMeth=Floor
  From Workspace : FromWorkspace  VariableName=Qh_noise  OutDataTypeStr=double  SampleTime=1500/fs
  From Workspace1 : FromWorkspace  VariableName=Ih_noise  OutDataTypeStr=double  SampleTime=1500/fs
  tlast : Constant  Value=0  SampleTime=1/fs
  tvalid : Constant  SampleTime=1/fs
  m_axis_tdata_imag : Outport
  m_axis_tdata_real : Outport  Port=2
  m_axis_tuser : Outport  Port=3
  m_axis_tvalid : Outport  Port=4
  m_axis_tlast : Outport  Port=5
  wires:
  Data Type Conversion6/1 -> Data Type Conversion5/1
  Data Type Conversion4/1 -> m_axis_tdata_imag/1
  Data Type Conversion8/1 -> Data Type Conversion4/1
  Data Type Conversion5/1 -> m_axis_tdata_real/1
  tvalid/1 -> m_axis_tvalid/1
  tlast/1 -> m_axis_tlast/1
  From Workspace/1 -> Buffer/1
  Buffer/1 -> Data Type Conversion8/1
  Buffer1/1 -> Data Type Conversion6/1
  From Workspace1/1 -> Buffer1/1
  Data Type Conversion2/1 -> Bit Concat1/1
  Constant1/1 -> Data Type Conversion2/1
  Constant/1 -> Data Type Conversion1/1
  Data Type Conversion1/1 -> Bit Concat1/2
  Bit Concat1/1 -> m_axis_tuser/1
